simulink model "EVdemo_6"  (R2013b)
settings: Solver=FixedStepDiscrete  SolverMode=SingleTasking  StartTime=0.0  StopTime=650  FixedStep=4e-5  MaxStep=1e-5  RelTol=1e-3
InitFcn:
  | %EV_Param_Update
  | % update the number of strings (discretized)
  | numStrings = round(Opti_numStrings);
  | %disp(['Number of strings: ' num2str(numStrings)])
  | % update the effective capacity based on the number of strings
  | EV_Param.Battery_Det.Rated_Capacity = 28.5*numStrings; %A*hr
  | EV_Param.Battery_Det.DP = 1.5*fliplr([1500 1500 1600 1450 1325 1125 925 675 425 175 ])./8*EV_Param.Battery_Det.Rated_Capacity; % 8 comes from the 8Ahr rated batter data used (normalize and rescale to the rated capacity
  | EV_Param.Battery_Det.CP = fliplr([25 100 200 250 375 550 750 950 1125 1150])./8*EV_Param.Battery_Det.Rated_Capacity;
  | 
  | % update the number of cells in a string (discretized)
  | numSeriesCells = round(Opti_numSeriesCells);
  | %disp(['Number of cells in a string: ' num2str(numSeriesCells)])
  | % update the nominal string volage and charge deficit
  | EV_Param.Battery_Det.Nominal_Voltage = numSeriesCells*cellVolts;
  | BatteryParams(1).Qe_init = 0;%EV_Param.Battery_Det.Rated_Capacity*(1-EV_Param.Battery_Det.Initial_SOC/100); %Ampere*hours
  | 
  | % update the total number of cells, battery pack mass and total vehicle
  | % mass
  | total_cells = numSeriesCells*numStrings;
  | %disp(['Total Number of cells: ' num2str(total_cells)])
  | EV_Param.BatteryMass = BatteryParams(1).cell_mass*total_cells;
  | %disp(['Total Battery Pack Mass: ' num2str(EV_Param.BatteryMass)])
  | EV_Param.Vehicle.Mass = 1300+EV_Param.BatteryMass;
  | 
  | % update the driveline gear ratio
  | EV_Param.Vehicle.Engine_Vehicle_Gear_Ratio = Opti_Vehicle_Gear_Ratio;
  | %disp(['Driveline gear ratio: ' num2str(Opti_Vehicle_Gear_Ratio)])
StartFcn:
  | %tic;
StopFcn:
  | %toc;
  | %disp([Final SOC: ' num2str(SOC_final)])
  | %disp([Final Vehicle Error: ' num2str(normed_SQE_final)])
model workspace (MAT data in the model file):
  MCOS : class17 (value not decoded)
  MCOS : class17 (value not decoded)
values from neighbouring files (symbols this model uses):
  Drive_Cycle_Num = 8    [startDemo.m]
undefined symbols (not defined in the file or in its folder): Acc_Cmd, BatteryParams, Brake_Set, cell_area, ctrlConst, current_phase_a, Dec_Cmd, direct_current, DiscIntNeverNeededParam, electromagnetic_torque, HEV_Param, Ion, Kt_Temps, Lithium, Mech_Power_kW, Opti_numSeriesCells, Opti_numStrings, Opti_Vehicle_Gear_Ratio, paramVelocityI, paramVelocityP, paramVelocityPICurrentSat, pmsm, quadrature_current, RLoadLoss, rotor_velocity, sigbuilder_block, Ts, Veh_Spd_Ref
libraries: fl_lib x306, nesl_utility x100, LeadAcidBattery_lib x60, simulink x23, powerlib x16, sdl_lib x7, elec_lib x4, electricdrivelib x2, checkpacklib x2, CustomDriveline_lib x2, LiBatteryBlocks x1, Capacitors_lib x1
(part 3 of 7)

== system EVdemo_6/DCDC_Converter/Detailed DC//DC Converter ==
  CBus : powerlib/Elements/Series RLC Branch  LConnTagsString=__new0  RConnTagsString=__new0  BranchType=RC  Resistance=0.1  Inductance=1e-3  SetiL0=off  InitialCurrent=0  Capacitance=1130e-6  Setx0=on  InitialVoltage=500  Measurements=None
  CBus1 : powerlib/Elements/Series RLC Branch  LConnTagsString=__new0  RConnTagsString=__new0  BranchType=C  Resistance=0.2  Inductance=1e-3  SetiL0=off  InitialCurrent=0  Capacitance=282e-6  Setx0=on  InitialVoltage=150  Measurements=None
  Detailed Boost converter : powerlib/Power Electronics/Universal Bridge  Arms=1  SnubberResistance=5000  SnubberCapacitance=inf  Device=IGBT / Diodes  Ron=1e-3  Lon=0  ForwardVoltages=[0,0]  ForwardVoltage=0  GTOparameters=[ 10e-6 , 20e-6 ]  IGBTparameters=[0,0]  Measurements=None  Measurements_2=None  converterType=Rectifier
  Ideal Heat Flow Source : fl_lib/Thermal/Thermal Sources/Ideal Heat Flow Source  Q_Log=off  T_Log=off  LocalVarNames=|heat_flow|T_differential  LocalVarDescs=|Heat flow through the source (J/s)|Temperature differential across the source (K)  LocalVarLogging=[0 0]
  L : powerlib/Elements/Series RLC Branch  LConnTagsString=__new0  RConnTagsString=__new0  BranchType=L  Resistance=0.3  Inductance=373e-6  SetiL0=off  InitialCurrent=100  Capacitance=100e-6  Setx0=off  InitialVoltage=0  Measurements=None
  PWM : Subsystem
  Simulink-PS Converter : nesl_utility/Simulink-PS Converter  PhysicalDomain=network_engine_domain  SubClassName=ps_input  LeftPortType=input  RightPortType=output  PseudoPeriodic=off  Frequencies=[]  NoiseDistribution=none  NoiseParameters=[]  Unit=1  AffineConversion=off  InputFiltering=off  SimscapeFilterOrder=1  InputFilterTimeConstant=0.001  UdotUserProvided=1
  Subsystem : Subsystem
      mask Display: disp('S');
  Subsystem1 : Subsystem
  Temperature Sensor : Subsystem
      mask Display:
      | patch([294.730220921338;294.546109275896;293.995547435362;293.083837611228;291.819760067491;290.215488561913;288.286473106077;286.051291173329;283.531468787557;280.75127321581;277.737479261253;274.519111407178;271.127164295357;267.594304230703;263.954554586898;260.242968142701;256.495289504528;252.747610866356;249.036024422158;245.396274778353;241.8634147137;238.471467601878;235.253099747803;232.239305793246;229.459110221499;226.939287835727;224.704105902979;222.775090447143;221.170818941565;219.906741397828;218.995031573694;218.44446973316;218.260358087718;218.44446973316;218.995031573694;219.906741397828;221.170818941565;222.775090447143;224.704105902979;226.939287835727;229.459110221499;232.239305793247;235.253099747803;238.471467601878;241.8634147137;245.396274778353;249.036024422158;252.747610866356;256.495289504528;260.242968142701;263.954554586898;267.594304230703;271.127164295357;274.519111407178;277.737479261253;280.75127321581;283.531468787557;286.051291173329;288.286473106077;290.215488561913;291.819760067491;293.083837611228;293.995547435362;294.546109275896;294.730220921338;294.730220921338], [122.389574535191;118.641895897019;114.930309452821;111.290559809016;107.757699744363;104.365752632541;101.147384778466;98.1335908239095;95.3533952521624;92.8335728663899;90.598390933642;88.6693754778057;87.0651039722279;85.8010264284914;84.8893166043572;84.3387547638233;84.1546431183815;84.3387547638233;84.8893166043572;85.8010264284914;87.0651039722279;88.6693754778058;90.598390933642;92.83357286639;95.3533952521625;98.1335908239095;101.147384778466;104.365752632541;107.757699744363;111.290559809016;114.930309452821;118.641895897019;122.389574535191;126.137253173364;129.848839617561;133.488589261366;137.02144932602;140.413396437841;143.631764291917;146.645558246473;149.42575381822;151.945576203992;154.18075813674;156.109773592576;157.714045098154;158.978122641891;159.889832466025;160.440394306559;160.624505952001;160.440394306559;159.889832466025;158.978122641891;157.714045098154;156.109773592576;154.18075813674;151.945576203992;149.42575381822;146.645558246473;143.631764291917;140.413396437841;137.02144932602;133.488589261366;129.848839617561;126.137253173364;122.389574535191;122.389574535191], [0;0;0])
      | plot([294.730220921338;294.546109275896;293.995547435362;293.083837611228;291.819760067491;290.215488561913;288.286473106077;286.051291173329;283.531468787557;280.75127321581;277.737479261253;274.519111407178;271.127164295357;267.594304230703;263.954554586898;260.242968142701;256.495289504528;252.747610866356;249.036024422158;245.396274778353;241.8634147137;238.471467601878;235.253099747803;232.239305793246;229.459110221499;226.939287835727;224.704105902979;222.775090447143;221.170818941565;219.906741397828;218.995031573694;218.44446973316;218.260358087718;218.44446973316;218.995031573694;219.906741397828;221.170818941565;222.775090447143;224.704105902979;226.939287835727;229.459110221499;232.239305793247;235.253099747803;238.471467601878;241.8634147137;245.396274778353;249.036024422158;252.747610866356;256.495289504528;260.242968142701;263.954554586898;267.594304230703;271.127164295357;274.519111407178;277.737479261253;280.75127321581;283.531468787557;286.051291173329;288.286473106077;290.215488561913;291.819760067491;293.083837611228;293.995547435362;294.546109275896;294.730220921338;294.730220921338], [122.389574535191;118.641895897019;114.930309452821;111.290559809016;107.757699744363;104.365752632541;101.147384778466;98.1335908239095;95.3533952521624;92.8335728663899;90.598390933642;88.6693754778057;87.0651039722279;85.8010264284914;84.8893166043572;84.3387547638233;84.1546431183815;84.3387547638233;84.8893166043572;85.8010264284914;87.0651039722279;88.6693754778058;90.598390933642;92.83357286639;95.3533952521625;98.1335908239095;101.147384778466;104.365752632541;107.757699744363;111.290559809016;114.930309452821;118.641895897019;122.389574535191;126.137253173364;129.848839617561;133.488589261366;137.02144932602;140.413396437841;143.631764291917;146.645558246473;149.42575381822;151.945576203992;154.18075813674;156.109773592576;157.714045098154;158.978122641891;159.889832466025;160.440394306559;160.624505952001;160.440394306559;159.889832466025;158.978122641891;157.714045098154;156.109773592576;154.18075813674;151.945576203992;149.42575381822;146.645558246473;143.631764291917;140.413396437841;137.02144932602;133.488589261366;129.848839617561;126.137253173364;122.389574535191;122.389574535191])
      | plot([243.771309033036;263.613159768283;263.613159768283;243.771309033036;243.771309033036], [438.410416245461;438.410416245461;112.4371541664;112.4371541664;438.410416245461])
      | plot([510.219018906355;0;0;510.219018906355;510.219018906355], [509.274168871343;509.274168871343;0;0;509.274168871343])
      | ;
      | %color('red');
      | %port_label('LConn', 1,'A')
      | %port_label('RConn', 1,'B')
  Thermal Mass : fl_lib/Thermal/Thermal Elements/Thermal Mass  mass=EV_Param.DCDCConv.Thermal_Mass kg  sp_heat=EV_Param.DCDCConv.Specific_Heat J/kg/K  init_temp=EV_Param.DCDCConv.Initial_Temperature C  Q_Log=off  LocalVarNames=|heat_flow|temperature  LocalVarDescs=|Heat flow (J/s)|Mass temperature (K)  LocalVarLogging=[0 0]
  Thermal Ref : fl_lib/Thermal/Thermal Elements/Thermal Reference  Q_Log=off  LocalVarNames=|Q  LocalVarDescs=|Q  LocalVarLogging=[]
  Ubus Ref : Constant  Value=HEV_Param.DCDCConv.Output_Voltage
  V1 : powerlib/Measurements/Voltage Measurement  PhasorSimulation=off  OutputType=Complex  PSBequivalent=0
  Voltage Controller : Subsystem  mask(PI controller){Kp=0.001, Ki=1, Ts=EV_Param.DCDCConv.Control_TS}
      mask prompts: Kp "Proportional gain (Kp)"; Ki "Integral gain (Ki)"; Ts "Sample time (s) :"
      mask help: Proportional-Integral Speed Controller
      mask Display: plot(0,0,100,100,[35,35,65],[70,30,30],[35,65],[45,60])
  Voltage-Current Simscape Interface : powerlib/Interface Elements/Voltage-Current Simscape Interface  DFT=off  Fmode=Low pass filter (continuous)  T=1e-6  Ts=50e-6  i0=0  v0=0  Sd=SimPowerSystems side  Measurements=off
  Voltage-Current Simscape Interface1 : powerlib/Interface Elements/Voltage-Current Simscape Interface  DFT=off  Fmode=Low pass filter (continuous)  T=1e-6  Ts=50e-6  i0=0  v0=0  Sd=SimPowerSystems side  Measurements=off
  " Batt+" : PMIOPort  Tag=PMCPort  Port=1  Side=Left
  " Batt-" : PMIOPort  Tag=PMCPort  Port=2  Side=Left
  " Bus+" : PMIOPort  Tag=PMCPort  Port=3  Side=Right
  " Bus-" : PMIOPort  Tag=PMCPort  Port=4  Side=Right
  H : PMIOPort  Tag=PMCPort  Port=5  Side=Right
  wires:
  V1/1 -> Voltage Controller/2(UBus)
  Ubus Ref/1 -> Voltage Controller/1(Uref)
  Voltage Controller/1(Ec) -> Subsystem1/1(IBus), PWM/1(Ref.)
  PWM/1(Pulses) -> Detailed Boost converter/1
  Subsystem1/1(Heat Flow) -> Simulink-PS Converter/1
  connections:
  Voltage-Current Simscape Interface1/LConn2 -- CBus/RConn1 -- V1/LConn2 -- Detailed Boost converter/RConn2 -- Voltage-Current Simscape Interface/LConn2 -- CBus1/RConn1
  CBus/LConn1 -- Voltage-Current Simscape Interface1/LConn1 -- V1/LConn1 -- Detailed Boost converter/RConn1
  L/LConn1 -- Detailed Boost converter/LConn1
  L/RConn1 -- Voltage-Current Simscape Interface/LConn1 -- CBus1/LConn1
  Voltage-Current Simscape Interface/RConn2 -- " Batt-"/RConn1
  " Batt+"/RConn1 -- Voltage-Current Simscape Interface/RConn1
  Voltage-Current Simscape Interface1/RConn1 -- " Bus+"/RConn1
  Voltage-Current Simscape Interface1/RConn2 -- " Bus-"/RConn1
  H/RConn1 -- Ideal Heat Flow Source/LConn1 -- Temperature Sensor/LConn1 -- Thermal Mass/LConn1
  Thermal Ref/LConn1 -- Ideal Heat Flow Source/RConn2
  Subsystem/RConn1 -- Ideal Heat Flow Source/RConn1
  Simulink-PS Converter/RConn1 -- Subsystem/LConn1

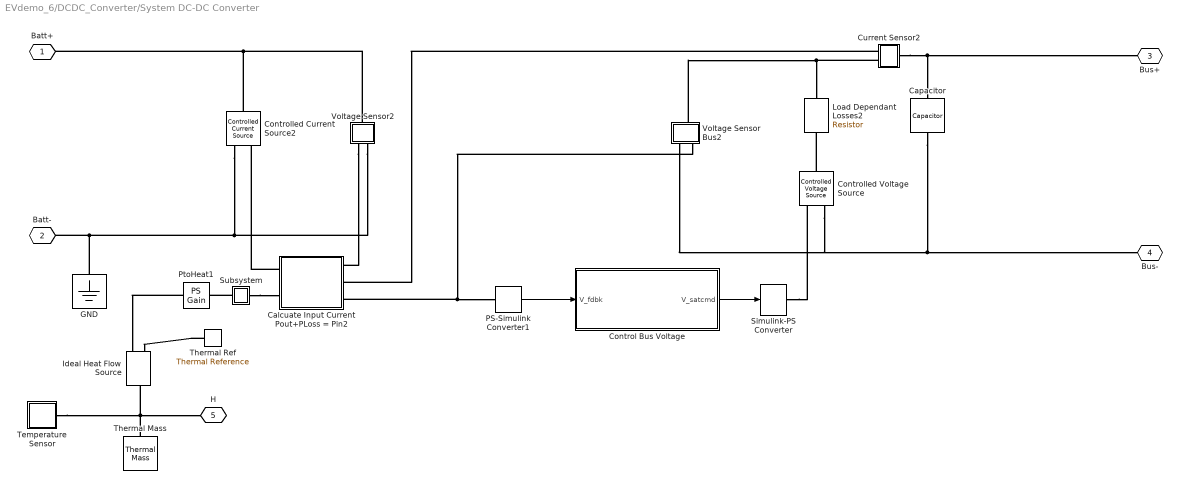
== system EVdemo_6/DCDC_Converter/System DC-DC Converter ==
  Calcuate Input Current Pout+PLoss = Pin2 : Subsystem
  Capacitor : fl_lib/Electrical/Electrical Elements/Capacitor  c=250e-6 F  v0=0 V  r=1e-6 Ohm  g=0 1/Ohm  i_Log=off  v_Log=off  vc_Log=off  LocalVarNames=|i|v|vc  LocalVarDescs=|i|v|Internal variable for voltage across capacitor term  LocalVarLogging=[0 0 0]
  Control Bus Voltage : Subsystem
  Controlled Current Source2 : fl_lib/Electrical/Electrical Sources/Controlled Current Source  i_Log=off  v_Log=off  LocalVarNames=|i|v  LocalVarDescs=|i|v  LocalVarLogging=[0 0]
  Controlled Voltage Source : fl_lib/Electrical/Electrical Sources/Controlled Voltage Source  i_Log=off  v_Log=off  LocalVarNames=|i|v  LocalVarDescs=|i|v  LocalVarLogging=[0 0]
  Current Sensor2 : Subsystem
  GND : fl_lib/Electrical/Electrical Elements/Electrical Reference  i_Log=off  LocalVarNames=|i  LocalVarDescs=|i  LocalVarLogging=0
  Ideal Heat Flow Source : fl_lib/Thermal/Thermal Sources/Ideal Heat Flow Source  Q_Log=off  T_Log=off  LocalVarNames=|heat_flow|T_differential  LocalVarDescs=|Heat flow through the source (J/s)|Temperature differential across the source (K)  LocalVarLogging=[0 0]
  Load Dependant Losses2 : fl_lib/Electrical/Electrical Elements/Resistor  R=RLoadLoss Ohm  i_Log=off  v_Log=off  LocalVarNames=|i|v  LocalVarDescs=|i|v  LocalVarLogging=[0 0]
  PS-Simulink Converter1 : nesl_utility/PS-Simulink Converter  PhysicalDomain=network_engine_domain  SubClassName=ps_output  LeftPortType=input  RightPortType=output  PseudoPeriodic=off  Frequencies=[]  Unit=1  AffineConversion=off
  PtoHeat1 : fl_lib/Physical Signals/Functions/PS Gain  gain=EV_Param.DCDCConv.EPower2Heat  LocalVarLogging=[]
  Simulink-PS Converter : nesl_utility/Simulink-PS Converter  PhysicalDomain=network_engine_domain  SubClassName=ps_input  LeftPortType=input  RightPortType=output  PseudoPeriodic=off  Frequencies=[]  NoiseDistribution=none  NoiseParameters=[]  Unit=1  AffineConversion=off  InputFiltering=off  SimscapeFilterOrder=1  InputFilterTimeConstant=0.001  UdotUserProvided=1
  Subsystem : Subsystem
      mask Display: disp('S');
  Temperature Sensor : Subsystem
      mask Display:
      | patch([294.730220921338;294.546109275896;293.995547435362;293.083837611228;291.819760067491;290.215488561913;288.286473106077;286.051291173329;283.531468787557;280.75127321581;277.737479261253;274.519111407178;271.127164295357;267.594304230703;263.954554586898;260.242968142701;256.495289504528;252.747610866356;249.036024422158;245.396274778353;241.8634147137;238.471467601878;235.253099747803;232.239305793246;229.459110221499;226.939287835727;224.704105902979;222.775090447143;221.170818941565;219.906741397828;218.995031573694;218.44446973316;218.260358087718;218.44446973316;218.995031573694;219.906741397828;221.170818941565;222.775090447143;224.704105902979;226.939287835727;229.459110221499;232.239305793247;235.253099747803;238.471467601878;241.8634147137;245.396274778353;249.036024422158;252.747610866356;256.495289504528;260.242968142701;263.954554586898;267.594304230703;271.127164295357;274.519111407178;277.737479261253;280.75127321581;283.531468787557;286.051291173329;288.286473106077;290.215488561913;291.819760067491;293.083837611228;293.995547435362;294.546109275896;294.730220921338;294.730220921338], [122.389574535191;118.641895897019;114.930309452821;111.290559809016;107.757699744363;104.365752632541;101.147384778466;98.1335908239095;95.3533952521624;92.8335728663899;90.598390933642;88.6693754778057;87.0651039722279;85.8010264284914;84.8893166043572;84.3387547638233;84.1546431183815;84.3387547638233;84.8893166043572;85.8010264284914;87.0651039722279;88.6693754778058;90.598390933642;92.83357286639;95.3533952521625;98.1335908239095;101.147384778466;104.365752632541;107.757699744363;111.290559809016;114.930309452821;118.641895897019;122.389574535191;126.137253173364;129.848839617561;133.488589261366;137.02144932602;140.413396437841;143.631764291917;146.645558246473;149.42575381822;151.945576203992;154.18075813674;156.109773592576;157.714045098154;158.978122641891;159.889832466025;160.440394306559;160.624505952001;160.440394306559;159.889832466025;158.978122641891;157.714045098154;156.109773592576;154.18075813674;151.945576203992;149.42575381822;146.645558246473;143.631764291917;140.413396437841;137.02144932602;133.488589261366;129.848839617561;126.137253173364;122.389574535191;122.389574535191], [0;0;0])
      | plot([294.730220921338;294.546109275896;293.995547435362;293.083837611228;291.819760067491;290.215488561913;288.286473106077;286.051291173329;283.531468787557;280.75127321581;277.737479261253;274.519111407178;271.127164295357;267.594304230703;263.954554586898;260.242968142701;256.495289504528;252.747610866356;249.036024422158;245.396274778353;241.8634147137;238.471467601878;235.253099747803;232.239305793246;229.459110221499;226.939287835727;224.704105902979;222.775090447143;221.170818941565;219.906741397828;218.995031573694;218.44446973316;218.260358087718;218.44446973316;218.995031573694;219.906741397828;221.170818941565;222.775090447143;224.704105902979;226.939287835727;229.459110221499;232.239305793247;235.253099747803;238.471467601878;241.8634147137;245.396274778353;249.036024422158;252.747610866356;256.495289504528;260.242968142701;263.954554586898;267.594304230703;271.127164295357;274.519111407178;277.737479261253;280.75127321581;283.531468787557;286.051291173329;288.286473106077;290.215488561913;291.819760067491;293.083837611228;293.995547435362;294.546109275896;294.730220921338;294.730220921338], [122.389574535191;118.641895897019;114.930309452821;111.290559809016;107.757699744363;104.365752632541;101.147384778466;98.1335908239095;95.3533952521624;92.8335728663899;90.598390933642;88.6693754778057;87.0651039722279;85.8010264284914;84.8893166043572;84.3387547638233;84.1546431183815;84.3387547638233;84.8893166043572;85.8010264284914;87.0651039722279;88.6693754778058;90.598390933642;92.83357286639;95.3533952521625;98.1335908239095;101.147384778466;104.365752632541;107.757699744363;111.290559809016;114.930309452821;118.641895897019;122.389574535191;126.137253173364;129.848839617561;133.488589261366;137.02144932602;140.413396437841;143.631764291917;146.645558246473;149.42575381822;151.945576203992;154.18075813674;156.109773592576;157.714045098154;158.978122641891;159.889832466025;160.440394306559;160.624505952001;160.440394306559;159.889832466025;158.978122641891;157.714045098154;156.109773592576;154.18075813674;151.945576203992;149.42575381822;146.645558246473;143.631764291917;140.413396437841;137.02144932602;133.488589261366;129.848839617561;126.137253173364;122.389574535191;122.389574535191])
      | plot([243.771309033036;263.613159768283;263.613159768283;243.771309033036;243.771309033036], [438.410416245461;438.410416245461;112.4371541664;112.4371541664;438.410416245461])
      | plot([510.219018906355;0;0;510.219018906355;510.219018906355], [509.274168871343;509.274168871343;0;0;509.274168871343])
      | ;
      | %color('red');
      | %port_label('LConn', 1,'A')
      | %port_label('RConn', 1,'B')
  Thermal Mass : fl_lib/Thermal/Thermal Elements/Thermal Mass  mass=EV_Param.DCDCConv.Thermal_Mass kg  sp_heat=EV_Param.DCDCConv.Specific_Heat J/kg/K  init_temp=EV_Param.DCDCConv.Initial_Temperature C  Q_Log=off  LocalVarNames=|heat_flow|temperature  LocalVarDescs=|Heat flow (J/s)|Mass temperature (K)  LocalVarLogging=[0 0]
  Thermal Ref : fl_lib/Thermal/Thermal Elements/Thermal Reference  Q_Log=off  LocalVarNames=|Q  LocalVarDescs=|Q  LocalVarLogging=[]
  Voltage Sensor Bus2 : Subsystem
  Voltage Sensor2 : Subsystem
  " Batt+" : PMIOPort  Tag=PMCPort  Port=1  Side=Left
  " Batt-" : PMIOPort  Tag=PMCPort  Port=2  Side=Left
  " Bus+" : PMIOPort  Tag=PMCPort  Port=3  Side=Right
  " Bus-" : PMIOPort  Tag=PMCPort  Port=4  Side=Right
  H : PMIOPort  Tag=PMCPort  Port=5  Side=Right
  wires:
  Control Bus Voltage/1(V_satcmd) -> Simulink-PS Converter/1
  PS-Simulink Converter1/1 -> Control Bus Voltage/1(V_fdbk)
  connections:
  Capacitor/RConn1 -- Voltage Sensor Bus2/RConn1 -- Controlled Voltage Source/RConn2 -- " Bus-"/RConn1
  Current Sensor2/LConn1 -- Capacitor/LConn1 -- " Bus+"/RConn1
  Controlled Current Source2/LConn1 -- Voltage Sensor2/LConn1 -- " Batt+"/RConn1
  Controlled Current Source2/RConn2 -- Voltage Sensor2/RConn2 -- GND/LConn1 -- " Batt-"/RConn1
  Voltage Sensor2/RConn1 -- Calcuate Input Current Pout+PLoss = Pin2/LConn1
  Calcuate Input Current Pout+PLoss = Pin2/RConn1 -- Controlled Current Source2/RConn1
  Subsystem/LConn1 -- Calcuate Input Current Pout+PLoss = Pin2/RConn2
  Controlled Voltage Source/LConn1 -- Load Dependant Losses2/RConn1
  Current Sensor2/RConn2 -- Voltage Sensor Bus2/LConn1 -- Load Dependant Losses2/LConn1
  Voltage Sensor Bus2/RConn2 -- PS-Simulink Converter1/LConn1 -- Calcuate Input Current Pout+PLoss = Pin2/LConn3
  Current Sensor2/RConn1 -- Calcuate Input Current Pout+PLoss = Pin2/LConn2
  Simulink-PS Converter/RConn1 -- Controlled Voltage Source/RConn1
  Thermal Ref/LConn1 -- Ideal Heat Flow Source/RConn2
  Subsystem/RConn1 -- PtoHeat1/LConn1
  PtoHeat1/RConn1 -- Ideal Heat Flow Source/RConn1
  Thermal Mass/LConn1 -- H/RConn1 -- Temperature Sensor/LConn1 -- Ideal Heat Flow Source/LConn1

== system EVdemo_6/Drive & Motor/Detailed_Motor ==
  System Inputs : Inport
  Continuous To Discrete1 : Subsystem
      mask Display: fprintf('C/D')
  Discrete To Continuous1 : Subsystem  Description=""
      mask Display: fprintf('D/C')
  Motor And Sensors : Subsystem
      mask Display: image('rtwdemo_pmsmfoc_motor.png')
  Velocity Controller : ModelReference  ModelNameDialog=PMSMvelocityController  SimulationMode=Normal  ModelReferenceVersion=1.84  CopyOfModelName=PMSMvelocityController  DefaultDataLogging=on
  ZZZ_Background_Box : Subsystem
      mask Display:
      | % text(0.5, 0.95,'Processor',...
      | %   'HorizontalAlignment', 'Center',...
      | %   'VerticalAlignment', 'Top',...
      | %   'texmode', 'on')
  + : PMIOPort  Port=1  Side=Left
  R : PMIOPort  Port=2  Side=Right
  - : PMIOPort  Port=3  Side=Left
  H : PMIOPort  Port=4  Side=Left
  Motor_Fdbk : Outport
  wires:
  Discrete To Continuous1/1(Motor Command) -> Motor And Sensors/1(Controller)
  Velocity Controller/1 -> Discrete To Continuous1/1(V)
  Continuous To Discrete1/4(Electrical Position) -> Velocity Controller/4
  Continuous To Discrete1/3(Phase Currents) -> Velocity Controller/3
  Continuous To Discrete1/1(Command) -> Velocity Controller/1
  Continuous To Discrete1/2(Rotor Velocity) -> Velocity Controller/2
  System Inputs/1 -> Continuous To Discrete1/1(System Inputs)
  Motor And Sensors/1(Motor_Fdbk) -> Continuous To Discrete1/2(Motor Measurements), Motor_Fdbk/1
  connections:
  +/RConn1 -- Motor And Sensors/LConn1
  -/RConn1 -- Motor And Sensors/LConn2
  Motor And Sensors/RConn1 -- R/RConn1
  H/RConn1 -- Motor And Sensors/LConn3

== system EVdemo_6/Drive & Motor/System_Motor ==
  System Inputs : Inport
  Continuous To Discrete1 : Subsystem
      mask Display: fprintf('C/D')
  Control_Velocity (Explicit_Ts) : Subsystem
      mask Display: fprintf('Control\nVelocity')
  Discrete To Continuous1 : Subsystem  Description=""
      mask Display: fprintf('D/C')
  Synchronous Motor & Drive : Subsystem
      mask Display:
      | image(imread('HEV_System_Motor_IMAGE.jpg'));
      | port_label('input',1,'T_Req');
      | port_label('LConn',1,'+');
      | port_label('LConn',2,'-');
      | port_label('RConn',1,'Shaft');
  ZZZ_Background_Box : Subsystem
      mask Display:
      | % text(0.5, 0.95,'Processor',...
      | %   'HorizontalAlignment', 'Center',...
      | %   'VerticalAlignment', 'Top',...
      | %   'texmode', 'on')
  + : PMIOPort  Port=1  Side=Left
  R : PMIOPort  Port=2  Side=Right
  - : PMIOPort  Port=3  Side=Left
  H : PMIOPort  Port=4  Side=Left
  Motor_Fdbk : Outport
  wires:
  Synchronous Motor & Drive/1(Fdbk) -> Motor_Fdbk/1, Continuous To Discrete1/2(Motor Measurements)
  Continuous To Discrete1/4(Rotor Velocity) -> Control_Velocity (Explicit_Ts)/4(velocity_measured)
  Control_Velocity (Explicit_Ts)/1(torque_cmd) -> Discrete To Continuous1/1(T)
  Discrete To Continuous1/1(Motor Command) -> Synchronous Motor & Drive/1(Cmd)
  Continuous To Discrete1/1(Command) -> Control_Velocity (Explicit_Ts)/1(velocity_command)
  System Inputs/1 -> Continuous To Discrete1/1(System Inputs)
  Continuous To Discrete1/2(Command1) -> Control_Velocity (Explicit_Ts)/2(mtr_torque_lim)
  Continuous To Discrete1/3(Command2) -> Control_Velocity (Explicit_Ts)/3(regen_torque_lim)
  connections:
  R/RConn1 -- Synchronous Motor & Drive/RConn1
  -/RConn1 -- Synchronous Motor & Drive/LConn2
  Synchronous Motor & Drive/LConn1 -- +/RConn1
  H/RConn1 -- Synchronous Motor & Drive/LConn3

== system EVdemo_6/Kph Demand/10-15 mode  ==
  Demux : Demux  Tag=STV Demux  Outputs=1
  FromWs : FromWorkspace  Tag=STV FromWs  VariableName=tuvar  SampleTime=0
      SigBuilderData=|
      | common.afterFinalStr = 'Extrapolate'
      | common.sampleTime = '0'
      | dataSet.timeRange = [0 660]
      | dataSet.name = '10-15 Mode Cycle'
      | sbobj.Groups.Name = '10-15 Mode Cycle'
      | sbobj.Groups.Signals.Name = 'Target speed'
      | sbobj.Groups.Signals.XData = [0 44 51 66 73 89 103 118 128 130 142 152 159 179 186 201 208 224 238 253 263 265 277 287 294 314 321 336 343 359 373 388 398 400 412 422 429 494 512 524 528 532 548 558 569 579 589 593 615 620 640 650 660]
      | sbobj.Groups.Signals.YData = [0 0 20 20 0 0 40 40 20 20 40 20 0 0 20 20 0 0 40 40 20 20 40 20 0 0 20 20 0 0 40 40 20 20 40 20 0 0 50 50 40 40 60 60 70 70 50 50 70 70 30 0 0]
  Target speed : Outport  Tag=STV Outport
  wires:
  Demux/1 -> Target speed/1
  FromWs/1 -> Demux/1

== system EVdemo_6/Motor & Power Managment/ZZZ_Background_Box ==

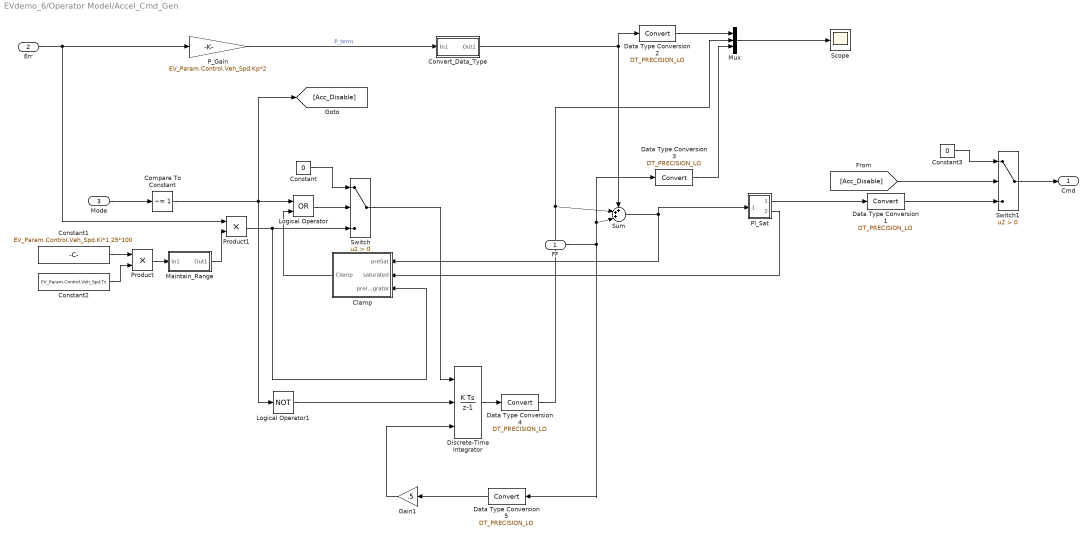
== system EVdemo_6/Operator Model/Accel_Cmd_Gen ==
  FF : Inport
  Err : Inport  Port=2
  Mode : Inport  Port=3
  Clamp : Subsystem
  Compare To Constant : simulink/Logic and Bit Operations/Compare To Constant  relop=~=  const=1  OutDataTypeStr=boolean
  Constant : Constant  Value=0  OutDataTypeStr=Inherit: Inherit via back propagation  SampleTime=-1  PreserveConstantTs=on
  Constant1 : Constant  Value=EV_Param.Control.Veh_Spd.Ki*1.25*100  SampleTime=-1
  Constant2 : Constant  Value=EV_Param.Control.Veh_Spd.Ts  OutDataTypeStr=DT_PRECISION_LO  SampleTime=-1
  Constant3 : Constant  Value=0  OutDataTypeStr=Inherit: Inherit via back propagation  SampleTime=-1  PreserveConstantTs=on
  Convert_Data_Type : Subsystem
      mask Display: fprintf('Double\nRange')
  Data Type Conversion{1..5} (5 alike) : DataTypeConversion  OutMin=-ctrlConst.CurrentMax  OutMax=ctrlConst.CurrentMax  OutDataTypeStr=DT_PRECISION_LO
      settings: AttributesFormatString=-----------------------------\nMin = %<OutMin>\nMax = %<OutMax>
  Discrete-Time Integrator : DiscreteIntegrator  ExternalReset=rising  InitialConditionSource=external  SampleTime=-1  ICPrevOutput=DiscIntNeverNeededParam  ICPrevScaledInput=DiscIntNeverNeededParam
  Gain1 : Gain  Gain=.5
  Logical Operator : Logic  Operator=OR  AllPortsSameDT=off  OutDataTypeStr=boolean
  Logical Operator1 : Logic  Operator=NOT  AllPortsSameDT=off  OutDataTypeStr=boolean
  Maintain_Range : Subsystem
      mask Display: fprintf('Maintain\nRange')
  Mux : Mux  Inputs=3
  PI_Sat : Subsystem
      mask Display: plot([0.15 0.85],[.5 .5],[.5 .5],[0.05 0.95],0.15+0.7*[0 .25 .75 1],0.05+0.9*[.25 .25 .75 .75]);
  P_Gain : Gain  Gain=EV_Param.Control.Veh_Spd.Kp*2  ParamDataTypeStr=Inherit: Inherit from 'Gain'
      settings: AttributesFormatString=-----------------------------\n%<Gain>
  Product : Product
  Product1 : Product
  Scope : Scope
      settings: YMin=-0.02  YMax=0.18  SaveName=ScopeData18
  Sum : Sum  Inputs=+++|
  Switch : Switch  Criteria=u2 > Threshold  InputSameDT=on
  Switch1 : Switch  Criteria=u2 > Threshold  InputSameDT=on
  Cmd : Outport
  wires:
  Convert_Data_Type/1(Out1) -> Sum/1, Data Type Conversion2/1
  PI_Sat/2(saturated) -> Clamp/2(saturated)
  Err/1 -> Product1/1, P_Gain/1
  P_Gain/1 -> Convert_Data_Type/1(In1)  "P_term"
  Constant/1 -> Switch/1
  Clamp/1(Clamp) -> Logical Operator/2
  Constant1/1 -> Product/1
  Constant2/1 -> Product/2
  Product/1 -> Maintain_Range/1(In1)
  Maintain_Range/1(Out1) -> Product1/2
  PI_Sat/1(Out1) -> Data Type Conversion1/1
  Data Type Conversion1/1 -> Switch1/3
  FF/1 -> Data Type Conversion5/1, Data Type Conversion3/1, Sum/3
  Data Type Conversion2/1 -> Mux/1
  Mux/1 -> Scope/1
  Data Type Conversion3/1 -> Mux/3
  Mode/1 -> Compare To Constant/1
  Logical Operator/1 -> Switch/2
  Compare To Constant/1 -> Logical Operator1/1, [Acc_Disable], Logical Operator/1
  Switch1/1 -> Cmd/1
  [Acc_Disable] -> Switch1/2
  Sum/1 -> PI_Sat/1(In1), Clamp/1(preSat)
  Product1/1 -> Clamp/3(preIntegrator), Switch/3
  Discrete-Time Integrator/1 -> Data Type Conversion4/1
  Data Type Conversion4/1 -> Mux/2, Sum/2
  Data Type Conversion5/1 -> Gain1/1
  Logical Operator1/1 -> Discrete-Time Integrator/2
  Switch/1 -> Discrete-Time Integrator/1
  Gain1/1 -> Discrete-Time Integrator/3
  Constant3/1 -> Switch1/1

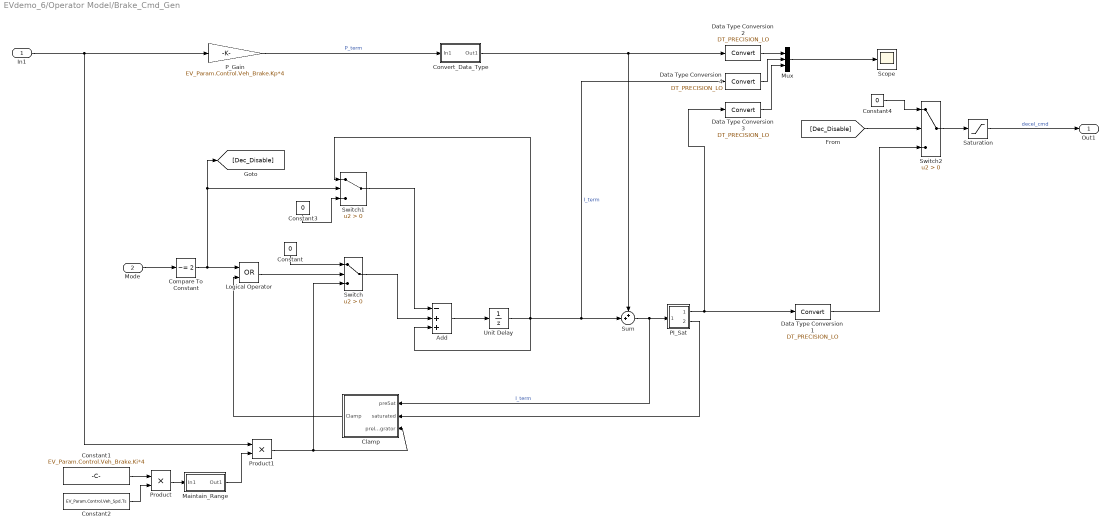
== system EVdemo_6/Operator Model/Brake_Cmd_Gen ==
  In1 : Inport
  Mode : Inport  Port=2
  Add : Sum  Inputs=-++  OutMin=-ctrlConst.CurrentMax*2  OutMax=ctrlConst.CurrentMax*2  OutDataTypeStr=DT_PRECISION_HI  SaturateOnIntegerOverflow=on
      settings: AttributesFormatString=-----------------------------\nMin = %<OutMin>\nMax = %<OutMax>\nSat = %<SaturateOnIntegerOverflow>
  Clamp : Subsystem
  Compare To Constant : simulink/Logic and Bit Operations/Compare To Constant  relop=~=  const=2  OutDataTypeStr=boolean
  Constant : Constant  Value=0  OutDataTypeStr=Inherit: Inherit via back propagation  SampleTime=-1  PreserveConstantTs=on
  Constant1 : Constant  Value=EV_Param.Control.Veh_Brake.Ki*4  SampleTime=-1
  Constant2 : Constant  Value=EV_Param.Control.Veh_Spd.Ts  OutDataTypeStr=DT_PRECISION_LO  SampleTime=-1
  Constant3 : Constant  Value=0  OutDataTypeStr=Inherit: Inherit via back propagation  SampleTime=-1  PreserveConstantTs=on
  Constant4 : Constant  Value=0  OutDataTypeStr=Inherit: Inherit via back propagation  SampleTime=-1  PreserveConstantTs=on
  Convert_Data_Type : Subsystem
      mask Display: fprintf('Double\nRange')
  Data Type Conversion{1..4} (4 alike) : DataTypeConversion  OutMin=-ctrlConst.CurrentMax  OutMax=ctrlConst.CurrentMax  OutDataTypeStr=DT_PRECISION_LO
      Data Type Conversion1 settings: AttributesFormatString=-----------------------------\nMin = %<OutMin>\nMax = %<OutMax>
  Logical Operator : Logic  Operator=OR  AllPortsSameDT=off  OutDataTypeStr=boolean
  Maintain_Range : Subsystem
      mask Display: fprintf('Maintain\nRange')
  Mux : Mux  Inputs=3
  PI_Sat : Subsystem
      mask Display: plot([0.15 0.85],[.5 .5],[.5 .5],[0.05 0.95],0.15+0.7*[0 .25 .75 1],0.05+0.9*[.25 .25 .75 .75]);
  P_Gain : Gain  Gain=EV_Param.Control.Veh_Brake.Kp*4  ParamDataTypeStr=Inherit: Inherit from 'Gain'
      settings: AttributesFormatString=-----------------------------\n%<Gain>
  Product : Product
  Product1 : Product
  Saturation : Saturate  UpperLimit=0  LowerLimit=-20
  Scope : Scope
      settings: YMin=-0.02  YMax=0.18  SaveName=ScopeData7
  Sum : Sum  Inputs=++|
  Switch : Switch  Criteria=u2 > Threshold  InputSameDT=on
  Switch1 : Switch  Criteria=u2 > Threshold  InputSameDT=on
  Switch2 : Switch  Criteria=u2 > Threshold  InputSameDT=on
  Unit Delay : UnitDelay  SampleTime=-1
  Out1 : Outport
  wires:
  Saturation/1 -> Out1/1  "decel_cmd"
  Data Type Conversion1/1 -> Switch2/3
  PI_Sat/1(Out1) -> Data Type Conversion1/1, Data Type Conversion3/1
  Maintain_Range/1(Out1) -> Product1/2
  Product/1 -> Maintain_Range/1(In1)
  Constant2/1 -> Product/2
  Constant1/1 -> Product/1
  Product1/1 -> Switch/3, Clamp/3(preIntegrator)
  Constant/1 -> Switch/1
  Unit Delay/1 -> Switch1/1, Data Type Conversion4/1, Sum/2, Add/3  "I_term"
  Add/1 -> Unit Delay/1
  P_Gain/1 -> Convert_Data_Type/1(In1)  "P_term"
  In1/1 -> Product1/1, P_Gain/1
  PI_Sat/2(saturated) -> Clamp/2(saturated)
  Switch/1 -> Add/2
  Convert_Data_Type/1(Out1) -> Sum/1, Data Type Conversion2/1
  Switch1/1 -> Add/1
  Constant3/1 -> Switch1/3
  Sum/1 -> Clamp/1(preSat), PI_Sat/1(In1)  "I_term"
  Data Type Conversion2/1 -> Mux/1
  Mux/1 -> Scope/1
  Data Type Conversion3/1 -> Mux/3
  Data Type Conversion4/1 -> Mux/2
  Mode/1 -> Compare To Constant/1
  Compare To Constant/1 -> [Dec_Disable], Switch1/2, Logical Operator/1
  Constant4/1 -> Switch2/1
  [Dec_Disable] -> Switch2/2
  Switch2/1 -> Saturation/1
  Logical Operator/1 -> Switch/2
  Clamp/1(Clamp) -> Logical Operator/2

== system EVdemo_6/Operator Model/LPF ==
  In : Inport
  Discrete-Time Integrator2 : DiscreteIntegrator  IntegratorMethod=Integration: Trapezoidal  SampleTime=-1  ShowStatePort=on  ICPrevOutput=DiscIntNeverNeededParam  ICPrevScaledInput=DiscIntNeverNeededParam
  FixPt Data Type Duplicate1 : DataTypeDuplicate  DisableCoverage=on  NumInputPorts=3
  Sum : Sum  Inputs=|+-
  w : Gain  Gain=w
  Out : Outport
  wires:
  Discrete-Time Integrator2/State -> Sum/2
  Sum/1 -> w/1
  Discrete-Time Integrator2/1 -> Out/1, FixPt Data Type Duplicate1/1
  In/1 -> Sum/1, FixPt Data Type Duplicate1/3
  w/1 -> Discrete-Time Integrator2/1, FixPt Data Type Duplicate1/2

== system EVdemo_6/Operator Model/LPF1 ==
  In : Inport
  Discrete-Time Integrator2 : DiscreteIntegrator  IntegratorMethod=Integration: Trapezoidal  SampleTime=-1  ShowStatePort=on  ICPrevOutput=DiscIntNeverNeededParam  ICPrevScaledInput=DiscIntNeverNeededParam
  FixPt Data Type Duplicate1 : DataTypeDuplicate  DisableCoverage=on  NumInputPorts=3
  Sum : Sum  Inputs=|+-
  w : Gain  Gain=w
  Out : Outport
  wires:
  w/1 -> FixPt Data Type Duplicate1/2, Discrete-Time Integrator2/1
  In/1 -> FixPt Data Type Duplicate1/3, Sum/1
  Discrete-Time Integrator2/1 -> FixPt Data Type Duplicate1/1, Out/1
  Sum/1 -> w/1
  Discrete-Time Integrator2/State -> Sum/2

== system EVdemo_6/Operator Model/delta_ref ==
  In1 : Inport
  Add : Sum  Inputs=+-
  Dead Zone : DeadZone  LowerValue=-0.1  UpperValue=0.1  SaturateOnIntegerOverflow=on
  Unit Delay : UnitDelay  SampleTime=-1
  Out1 : Outport
  wires:
  Unit Delay/1 -> Add/2
  Add/1 -> Dead Zone/1
  In1/1 -> Unit Delay/1, Add/1
  Dead Zone/1 -> Out1/1

== system EVdemo_6/System Analysis/0 to 60 Latch ==
  In1 : Inport
  Add1 : Sum
  Clock : Clock
  Compare To Constant : simulink/Logic and Bit Operations/Compare To Constant  relop=>=  const=97  OutDataTypeStr=boolean
  Constant1 : Constant  Value=0  SampleTime=-1
  Rate Transition : RateTransition
  Switch : Switch  Criteria=u2 > Threshold
  Switch1 : Switch  Criteria=u2 > Threshold
  Unit Delay : UnitDelay  SampleTime=-1
  Unit Delay1 : UnitDelay  SampleTime=-1
  Out1 : Outport
  wires:
  Clock/1 -> Rate Transition/1
  Switch1/1 -> Unit Delay1/1
  Constant1/1 -> Switch/1
  Unit Delay/1 -> Add1/2, Switch/2
  Unit Delay1/1 -> Out1/1, Switch1/1
  Switch/1 -> Add1/1
  Add1/1 -> Switch1/2, Unit Delay/1
  In1/1 -> Compare To Constant/1
  Rate Transition/1 -> Switch1/3
  Compare To Constant/1 -> Switch/3

== system EVdemo_6/System Analysis/Convert Rotor Velocity Units ==
  note: Convert Rotor Velocity Units
  note: Convert velocity units from radians per second to revolutions per minute.
  system_inputs : Inport
  system_measurements : Inport  Port=2
  Bus Creator1 : BusCreator  Inputs=2
  Bus Selector1 : BusSelector  OutputSignals=Motor_Fdbk.rotor_velocity
  Bus Selector2 : BusSelector  OutputSignals=Motor_Cmds.Motor_Spd_Ref_radps
  rad_per_sec_to_rpm_command : Gain  Gain=30/pi  OutDataTypeStr=double
  rad_per_sec_to_rpm_measured : Gain  Gain=30/pi
  rotor_velocities : Outport
  wires:
  Bus Selector2/1 -> rad_per_sec_to_rpm_command/1  "<Motor_Spd_Ref_radps>"
  Bus Selector1/1 -> rad_per_sec_to_rpm_measured/1  "<rotor_velocity>"
  Bus Creator1/1 -> rotor_velocities/1  "rotor_velocities"
  system_inputs/1 -> Bus Selector2/1
  system_measurements/1 -> Bus Selector1/1
  rad_per_sec_to_rpm_command/1 -> Bus Creator1/1  "rotor_ref_rpm"
  rad_per_sec_to_rpm_measured/1 -> Bus Creator1/2  "rotor_velocity_rpm"

== system EVdemo_6/Thermal_Partition/Battery Cold Plate ==
  Cold_Plate : fl_lib/Thermal/Thermal Elements/Conductive Heat Transfer  area=cell_area*2 m^2  thickness=0.005 m  th_cond=401 W/(m*K)  Q_Log=off  T_Log=off  LocalVarNames=|Q|T  LocalVarDescs=|Q|T  LocalVarLogging=[0 0]
  Ideal Heat Flow Sensor : fl_lib/Thermal/Thermal Sensors/Ideal Heat Flow Sensor  Q_Log=off  T_Log=off  LocalVarNames=|Q|T  LocalVarDescs=|Q|T  LocalVarLogging=[0 0]
  Ideal Heat Flow Source : fl_lib/Thermal/Thermal Sources/Ideal Heat Flow Source  Q_Log=off  T_Log=off  LocalVarNames=|Q|T  LocalVarDescs=|Q|T  LocalVarLogging=[0 0]
  Ideal Temperature Sensor : fl_lib/Thermal/Thermal Sensors/Ideal Temperature Sensor  Qs_Log=off  Ts_Log=off  LocalVarNames=|Qs|Ts  LocalVarDescs=|Qs|Ts  LocalVarLogging=[0 0]
  Ideal Temperature Source : fl_lib/Thermal/Thermal Sources/Ideal Temperature Source  Q_Log=off  T_Log=off  LocalVarNames=|Q|T  LocalVarDescs=|Q|T  LocalVarLogging=[0 0]
  PS-Simulink Converter1 : nesl_utility/PS-Simulink Converter  PhysicalDomain=network_engine_domain  SubClassName=ps_output  LeftPortType=input  RightPortType=output  PseudoPeriodic=off  Frequencies=[]  Unit=W  AffineConversion=on
  PS-Simulink Converter2 : nesl_utility/PS-Simulink Converter  PhysicalDomain=network_engine_domain  SubClassName=ps_output  LeftPortType=input  RightPortType=output  PseudoPeriodic=off  Frequencies=[]  Unit=K  AffineConversion=on
  Rate Transition : RateTransition
  Rate Transition1 : RateTransition  X0=BatteryParams(1).T_init
  Simulink-PS Converter : nesl_utility/Simulink-PS Converter  PhysicalDomain=network_engine_domain  SubClassName=ps_input  LeftPortType=input  RightPortType=output  PseudoPeriodic=off  Frequencies=[]  NoiseDistribution=none  NoiseParameters=[]  Unit=K  AffineConversion=on  InputFiltering=off  SimscapeFilterOrder=1  InputFilterTimeConstant=0.001  UdotUserProvided=1
  Simulink-PS Converter1 : nesl_utility/Simulink-PS Converter  PhysicalDomain=network_engine_domain  SubClassName=ps_input  LeftPortType=input  RightPortType=output  PseudoPeriodic=off  Frequencies=[]  NoiseDistribution=none  NoiseParameters=[]  Unit=W  AffineConversion=on  InputFiltering=off  SimscapeFilterOrder=1  InputFilterTimeConstant=0.001  UdotUserProvided=1
  Thermal Reference2 : fl_lib/Thermal/Thermal Elements/Thermal Reference  Q_Log=off  LocalVarNames=|Q  LocalVarDescs=|Q  LocalVarLogging=[]
  Thermal Reference3 : fl_lib/Thermal/Thermal Elements/Thermal Reference  Q_Log=off  LocalVarNames=|Q  LocalVarDescs=|Q  LocalVarLogging=[]
  Thermal Reference4 : fl_lib/Thermal/Thermal Elements/Thermal Reference  Q_Log=off  LocalVarNames=|Q  LocalVarDescs=|Q  LocalVarLogging=[]
  Thermal_Divider : Gain  Gain=1/total_cells
  Coolant_Port : PMIOPort  Port=1  Side=Right
  Electronic_Port : PMIOPort  Port=2  Side=Left
  wires:
  Rate Transition1/1 -> Simulink-PS Converter/1
  Thermal_Divider/1 -> Simulink-PS Converter1/1
  PS-Simulink Converter1/1 -> Rate Transition/1
  PS-Simulink Converter2/1 -> Rate Transition1/1
  Rate Transition/1 -> Thermal_Divider/1
  connections:
  Thermal Reference3/LConn1 -- Ideal Temperature Source/RConn2
  Ideal Temperature Sensor/RConn1 -- Thermal Reference2/LConn1
  Ideal Heat Flow Sensor/RConn2 -- Coolant_Port/RConn1
  Cold_Plate/RConn1 -- Ideal Heat Flow Sensor/LConn1
  Cold_Plate/LConn1 -- Ideal Temperature Source/LConn1
  Ideal Heat Flow Sensor/RConn1 -- PS-Simulink Converter1/LConn1
  Simulink-PS Converter/RConn1 -- Ideal Temperature Source/RConn1
  Ideal Temperature Sensor/RConn2 -- PS-Simulink Converter2/LConn1
  Thermal Reference4/LConn1 -- Ideal Heat Flow Source/LConn1
  Ideal Temperature Sensor/LConn1 -- Electronic_Port/RConn1 -- Ideal Heat Flow Source/RConn2
  Ideal Heat Flow Source/RConn1 -- Simulink-PS Converter1/RConn1

== system EVdemo_6/Thermal_Partition/DCDC Cold Plate ==
  Add : Sum  Inputs=+-
  Cold_Plate : fl_lib/Thermal/Thermal Elements/Conductive Heat Transfer  area=.1*.3 m^2  thickness=0.005 m  th_cond=401 W/(m*K)  Q_Log=off  T_Log=off  LocalVarNames=|Q|T  LocalVarDescs=|Q|T  LocalVarLogging=[0 0]
  Constant : Constant  Value=272.15  SampleTime=-1
  Ideal Heat Flow Sensor : fl_lib/Thermal/Thermal Sensors/Ideal Heat Flow Sensor  Q_Log=off  T_Log=off  LocalVarNames=|Q|T  LocalVarDescs=|Q|T  LocalVarLogging=[0 0]
  Ideal Heat Flow Source : fl_lib/Thermal/Thermal Sources/Ideal Heat Flow Source  Q_Log=off  T_Log=off  LocalVarNames=|Q|T  LocalVarDescs=|Q|T  LocalVarLogging=[0 0]
  Ideal Temperature Sensor : fl_lib/Thermal/Thermal Sensors/Ideal Temperature Sensor  Qs_Log=off  Ts_Log=off  LocalVarNames=|Qs|Ts  LocalVarDescs=|Qs|Ts  LocalVarLogging=[0 0]
  Ideal Temperature Source : fl_lib/Thermal/Thermal Sources/Ideal Temperature Source  Q_Log=off  T_Log=off  LocalVarNames=|Q|T  LocalVarDescs=|Q|T  LocalVarLogging=[0 0]
  PS-Simulink Converter1 : nesl_utility/PS-Simulink Converter  PhysicalDomain=network_engine_domain  SubClassName=ps_output  LeftPortType=input  RightPortType=output  PseudoPeriodic=off  Frequencies=[]  Unit=W  AffineConversion=on
  PS-Simulink Converter2 : nesl_utility/PS-Simulink Converter  PhysicalDomain=network_engine_domain  SubClassName=ps_output  LeftPortType=input  RightPortType=output  PseudoPeriodic=off  Frequencies=[]  Unit=K  AffineConversion=on
  Rate Transition : RateTransition
  Rate Transition1 : RateTransition  X0=BatteryParams(1).T_init
  Simulink-PS Converter : nesl_utility/Simulink-PS Converter  PhysicalDomain=network_engine_domain  SubClassName=ps_input  LeftPortType=input  RightPortType=output  PseudoPeriodic=off  Frequencies=[]  NoiseDistribution=none  NoiseParameters=[]  Unit=K  AffineConversion=on  InputFiltering=off  SimscapeFilterOrder=1  InputFilterTimeConstant=0.001  UdotUserProvided=1
  Simulink-PS Converter1 : nesl_utility/Simulink-PS Converter  PhysicalDomain=network_engine_domain  SubClassName=ps_input  LeftPortType=input  RightPortType=output  PseudoPeriodic=off  Frequencies=[]  NoiseDistribution=none  NoiseParameters=[]  Unit=W  AffineConversion=on  InputFiltering=off  SimscapeFilterOrder=1  InputFilterTimeConstant=0.001  UdotUserProvided=1
  Thermal Reference2 : fl_lib/Thermal/Thermal Elements/Thermal Reference  Q_Log=off  LocalVarNames=|Q  LocalVarDescs=|Q  LocalVarLogging=[]
  Thermal Reference3 : fl_lib/Thermal/Thermal Elements/Thermal Reference  Q_Log=off  LocalVarNames=|Q  LocalVarDescs=|Q  LocalVarLogging=[]
  Thermal Reference4 : fl_lib/Thermal/Thermal Elements/Thermal Reference  Q_Log=off  LocalVarNames=|Q  LocalVarDescs=|Q  LocalVarLogging=[]
  Coolant_Port : PMIOPort  Port=1  Side=Right
  Electronic_Port : PMIOPort  Port=2  Side=Left
  tag scope: DCDC_Temp=global
  wires:
  Rate Transition1/1 -> Simulink-PS Converter/1
  Rate Transition/1 -> Simulink-PS Converter1/1
  PS-Simulink Converter1/1 -> Rate Transition/1
  PS-Simulink Converter2/1 -> Add/1, Rate Transition1/1
  Constant/1 -> Add/2
  Add/1 -> [DCDC_Temp]
  connections:
  Ideal Temperature Sensor/LConn1 -- Electronic_Port/RConn1 -- Ideal Heat Flow Source/RConn2
  Thermal Reference3/LConn1 -- Ideal Temperature Source/RConn2
  Ideal Temperature Sensor/RConn1 -- Thermal Reference2/LConn1
  Ideal Heat Flow Sensor/RConn2 -- Coolant_Port/RConn1
  Cold_Plate/RConn1 -- Ideal Heat Flow Sensor/LConn1
  Cold_Plate/LConn1 -- Ideal Temperature Source/LConn1
  Ideal Heat Flow Sensor/RConn1 -- PS-Simulink Converter1/LConn1
  Ideal Heat Flow Source/RConn1 -- Simulink-PS Converter1/RConn1
  Simulink-PS Converter/RConn1 -- Ideal Temperature Source/RConn1
  Ideal Temperature Sensor/RConn2 -- PS-Simulink Converter2/LConn1
  Thermal Reference4/LConn1 -- Ideal Heat Flow Source/LConn1

== system EVdemo_6/Thermal_Partition/PMSM Cold Plate ==
  Add : Sum  Inputs=+-
  Cold_Plate : fl_lib/Thermal/Thermal Elements/Conductive Heat Transfer  area=.1*.3 m^2  thickness=0.005 m  th_cond=401 W/(m*K)  Q_Log=off  T_Log=off  LocalVarNames=|Q|T  LocalVarDescs=|Q|T  LocalVarLogging=[0 0]
  Constant : Constant  Value=272.15  SampleTime=-1
  Ideal Heat Flow Sensor : fl_lib/Thermal/Thermal Sensors/Ideal Heat Flow Sensor  Q_Log=off  T_Log=off  LocalVarNames=|Q|T  LocalVarDescs=|Q|T  LocalVarLogging=[0 0]
  Ideal Heat Flow Source : fl_lib/Thermal/Thermal Sources/Ideal Heat Flow Source  Q_Log=off  T_Log=off  LocalVarNames=|Q|T  LocalVarDescs=|Q|T  LocalVarLogging=[0 0]
  Ideal Temperature Sensor : fl_lib/Thermal/Thermal Sensors/Ideal Temperature Sensor  Qs_Log=off  Ts_Log=off  LocalVarNames=|Qs|Ts  LocalVarDescs=|Qs|Ts  LocalVarLogging=[0 0]
  Ideal Temperature Source : fl_lib/Thermal/Thermal Sources/Ideal Temperature Source  Q_Log=off  T_Log=off  LocalVarNames=|Q|T  LocalVarDescs=|Q|T  LocalVarLogging=[0 0]
  PS-Simulink Converter1 : nesl_utility/PS-Simulink Converter  PhysicalDomain=network_engine_domain  SubClassName=ps_output  LeftPortType=input  RightPortType=output  PseudoPeriodic=off  Frequencies=[]  Unit=W  AffineConversion=on
  PS-Simulink Converter2 : nesl_utility/PS-Simulink Converter  PhysicalDomain=network_engine_domain  SubClassName=ps_output  LeftPortType=input  RightPortType=output  PseudoPeriodic=off  Frequencies=[]  Unit=K  AffineConversion=on
  Rate Transition : RateTransition
  Rate Transition1 : RateTransition  X0=BatteryParams(1).T_init
  Simulink-PS Converter : nesl_utility/Simulink-PS Converter  PhysicalDomain=network_engine_domain  SubClassName=ps_input  LeftPortType=input  RightPortType=output  PseudoPeriodic=off  Frequencies=[]  NoiseDistribution=none  NoiseParameters=[]  Unit=K  AffineConversion=on  InputFiltering=off  SimscapeFilterOrder=1  InputFilterTimeConstant=0.001  UdotUserProvided=1
  Simulink-PS Converter1 : nesl_utility/Simulink-PS Converter  PhysicalDomain=network_engine_domain  SubClassName=ps_input  LeftPortType=input  RightPortType=output  PseudoPeriodic=off  Frequencies=[]  NoiseDistribution=none  NoiseParameters=[]  Unit=W  AffineConversion=on  InputFiltering=off  SimscapeFilterOrder=1  InputFilterTimeConstant=0.001  UdotUserProvided=1
  Thermal Reference2 : fl_lib/Thermal/Thermal Elements/Thermal Reference  Q_Log=off  LocalVarNames=|Q  LocalVarDescs=|Q  LocalVarLogging=[]
  Thermal Reference3 : fl_lib/Thermal/Thermal Elements/Thermal Reference  Q_Log=off  LocalVarNames=|Q  LocalVarDescs=|Q  LocalVarLogging=[]
  Thermal Reference4 : fl_lib/Thermal/Thermal Elements/Thermal Reference  Q_Log=off  LocalVarNames=|Q  LocalVarDescs=|Q  LocalVarLogging=[]
  Coolant_Port : PMIOPort  Port=1  Side=Right
  Electronic_Port : PMIOPort  Port=2  Side=Left
  tag scope: PMSM_Temp=global
  wires:
  PS-Simulink Converter1/1 -> Rate Transition/1
  Rate Transition/1 -> Simulink-PS Converter1/1
  Rate Transition1/1 -> Simulink-PS Converter/1
  PS-Simulink Converter2/1 -> Add/1, Rate Transition1/1
  Constant/1 -> Add/2
  Add/1 -> [PMSM_Temp]
  connections:
  Thermal Reference4/LConn1 -- Ideal Heat Flow Source/LConn1
  Ideal Temperature Sensor/RConn2 -- PS-Simulink Converter2/LConn1
  Simulink-PS Converter/RConn1 -- Ideal Temperature Source/RConn1
  Ideal Heat Flow Source/RConn1 -- Simulink-PS Converter1/RConn1
  Ideal Heat Flow Sensor/RConn1 -- PS-Simulink Converter1/LConn1
  Cold_Plate/LConn1 -- Ideal Temperature Source/LConn1
  Cold_Plate/RConn1 -- Ideal Heat Flow Sensor/LConn1
  Ideal Heat Flow Sensor/RConn2 -- Coolant_Port/RConn1
  Ideal Temperature Sensor/RConn1 -- Thermal Reference2/LConn1
  Thermal Reference3/LConn1 -- Ideal Temperature Source/RConn2
  Ideal Heat Flow Source/RConn2 -- Ideal Temperature Sensor/LConn1 -- Electronic_Port/RConn1
